simulink model "dahlinsim"  (R2018a)
settings: Solver=VariableStepAuto  StartTime=0.0  StopTime=10.0  RelTol=1e-3
settings Model: Creator=GRENTOR  LastModifiedBy=GRENTOR

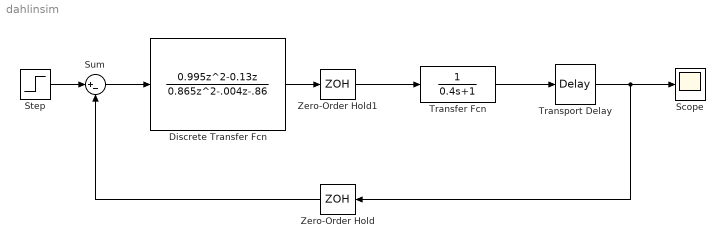
== system dahlinsim ==
  Discrete Transfer Fcn : DiscreteTransferFcn  Numerator=[0.995 -0.13 0]  Denominator="[0.865  -.004  -.86 ]"  SampleTime=0.8
  Scope : Scope
  Step : Step  SampleTime=0.8
  Sum : Sum  Inputs=|+-
  Transfer Fcn : TransferFcn  Denominator=[0.4 1]
  Transport Delay : TransportDelay  DelayTime=.8  FixedBuffer=on  PadeOrder=1
  Zero-Order Hold : ZeroOrderHold  SampleTime=0.8
  Zero-Order Hold1 : ZeroOrderHold  SampleTime=0.8
  wires:
  Zero-Order Hold/1 -> Sum/2
  Step/1 -> Sum/1
  Sum/1 -> Discrete Transfer Fcn/1
  Discrete Transfer Fcn/1 -> Zero-Order Hold1/1
  Zero-Order Hold1/1 -> Transfer Fcn/1
  Transfer Fcn/1 -> Transport Delay/1
  Transport Delay/1 -> Zero-Order Hold/1, Scope/1
